simulink model "HIL_version22b"  (R2022b)
settings: Solver=ode3  StartTime=0.0  StopTime=inf  FixedStep=0.01  RelTol=1e-3  EnableMultiTasking=on
undefined symbols (not defined in the file): K
libraries: arduinolib x3, simulink_extras x2, arduinosensorlib x1
settings Model: SimulationMode=external  ExtModeTrigDuration=2  Creator=Shehab Abdo  LastModifiedBy=Shehab Abdo
settings SolverCC: AutoInsertRateTranBlk=on
settings OptimizationCC: ReuseModelBlockBuffer=on  EnhancedBackFolding=on  PassReuseOutputArgsAs=Individual arguments  ZeroExternalMemoryAtStartup=off  ZeroInternalMemoryAtStartup=off  MaxStackSize=64  OptimizeBlockOrder=speed  DifferentSizesBufferReuse=on  OptimizationCustomize=off  EfficientTunableParamExpr=on
settings DebuggingCC: MultiTaskRateTransMsg=warning  ParameterTunabilityLossMsg=error
settings HardwareCC: ProdBitPerInt=16  ProdBitPerPointer=16  ProdBitPerSizeT=16  ProdBitPerPtrDiffT=16  ProdLargestAtomicFloat=None  ProdWordSize=8  ProdHWDeviceType=Atmel->AVR
settings SFSimCC: MATLABDynamicMemAlloc=off
settings RTWCC: Description=Embedded Coder  SystemTargetFile=ert.tlc  HardwareBoard=Arduino Mega 2560  TLCOptions=-aInlineSetEventsForThisBaseRateFcn=TLC_FALSE -aSuppressMultiTaskScheduler=TLC_FALSE -aRateBasedStepFcn=1  TemplateMakefile=ert_default_tmf  Toolchain=Arduino AVR  BuildConfiguration=Faster Runs
settings CodeAppCC: ForceParamTrailComments=on  IgnoreCustomStorageClasses=off  OperatorAnnotations=on  SimulinkDataObjDesc=on  SFDataObjDesc=on  InsertBlockDesc=on
settings ERTTargetCC: SupportContinuousTime=on  SupportVariableSizeSignals=on  ExtModeTransport=3  ExtModeStaticAlloc=on  ExtModeAutomaticAllocSize=off  ExtModeStaticAllocSize=2048  ExtModeMexFile=ext_xcp  ExtModeIntrfLevel=Level2 - Open

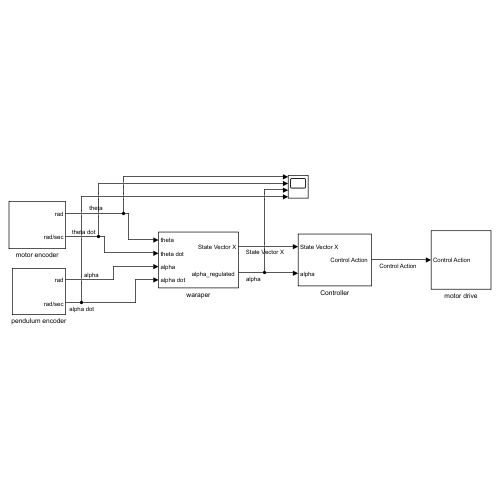
[thumbnail: Simulink's stored preview of the top-level diagram]
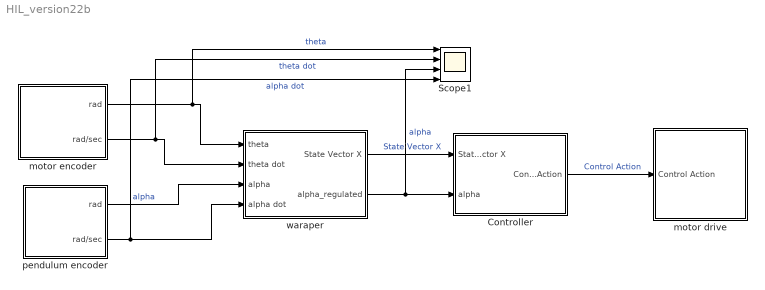
== system HIL_version22b ==
  Controller : Subsystem
  Scope1 : Scope  NumInputPorts=4
  motor drive : Subsystem
  motor encoder : Subsystem
  pendulum encoder : Subsystem
  waraper : Subsystem
  wires:
  Controller/1("Control Action ") -> motor drive/1(Control Action)  "Control Action"
  waraper/2("alpha_regulated ") -> Scope1/3, Controller/2(alpha)  "alpha"
  pendulum encoder/1(rad) -> waraper/3(alpha)  "alpha"
  motor encoder/2(rad/sec) -> Scope1/2, waraper/2(theta dot)  "theta dot"
  waraper/1(State Vector X) -> Controller/1(State Vector X)  "State Vector X"
  motor encoder/1(rad) -> Scope1/1, waraper/1(theta)  "theta"
  pendulum encoder/2(rad/sec) -> waraper/4(alpha dot), Scope1/4  "alpha dot"

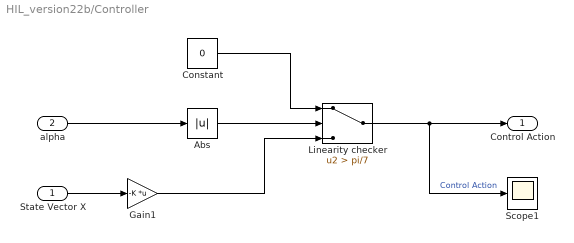
== system HIL_version22b/Controller ==
  State Vector X : Inport
  alpha : Inport  Port=2
  Abs : Abs  SaturateOnIntegerOverflow=off
  Constant : Constant  Value=0
  Gain1 : Gain  Gain=-K  Multiplication=Matrix(K*u)
  Linearity checker : Switch  Criteria=u2 > Threshold  Threshold=pi/7  SaturateOnIntegerOverflow=off  InputSameDT=off
  Scope1 : Scope
  "Control Action " : Outport
  wires:
  State Vector X/1 -> Gain1/1
  Constant/1 -> Linearity checker/1
  Linearity checker/1 -> "Control Action "/1, Scope1/1  "Control Action"
  Gain1/1 -> Linearity checker/3
  Abs/1 -> Linearity checker/2
  alpha/1 -> Abs/1

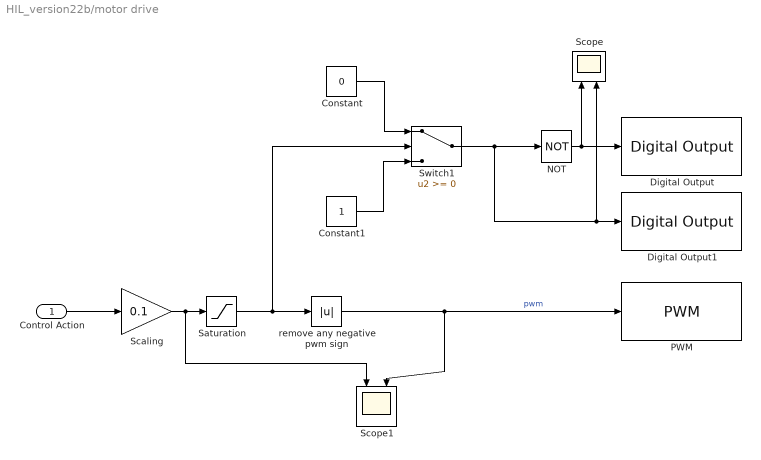
== system HIL_version22b/motor drive ==
  Control Action : Inport
  Constant : Constant  Value=0
  Constant1 : Constant
  Digital Output : arduinolib/Digital Output  pinNumber=7  Direction=output  blockPlatform=arduino
  Digital Output1 : arduinolib/Digital Output  pinNumber=8  Direction=output  blockPlatform=arduino
  NOT : Logic  Operator=NOT  IconShape=distinctive  AllPortsSameDT=off  OutDataTypeStr=boolean
  PWM : arduinolib/PWM  pinNumber=6  frequencyType=Default  desiredFrequency=490.2  achievableFrequency=490.2
  Saturation : Saturate  UpperLimit=255  LowerLimit=-255
  Scaling : Gain  Gain=0.1
  Scope : Scope  NumInputPorts=2
  Scope1 : Scope  NumInputPorts=2
  Switch1 : Switch  SaturateOnIntegerOverflow=off  InputSameDT=off
  remove any negative pwm sign : Abs  SaturateOnIntegerOverflow=off
  wires:
  remove any negative pwm sign/1 -> PWM/1, Scope1/2  "pwm"
  Saturation/1 -> Switch1/2, remove any negative pwm sign/1
  Constant/1 -> Switch1/1
  Control Action/1 -> Scaling/1
  Scaling/1 -> Scope1/1, Saturation/1
  Constant1/1 -> Switch1/3
  Switch1/1 -> Digital Output1/1, Scope/2, NOT/1
  NOT/1 -> Digital Output/1, Scope/1

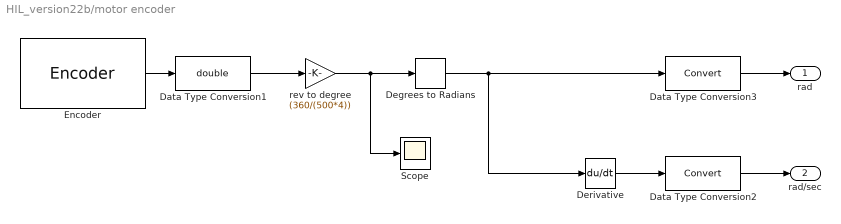
== system HIL_version22b/motor encoder ==
  Data Type Conversion1 : DataTypeConversion  OutDataTypeStr=double  SaturateOnIntegerOverflow=off  RndMeth=Floor
  Data Type Conversion2 : DataTypeConversion  SaturateOnIntegerOverflow=off  RndMeth=Floor
  Data Type Conversion3 : DataTypeConversion  SaturateOnIntegerOverflow=off  RndMeth=Floor
  Degrees to Radians : simulink_extras/Transformations/Degrees to Radians
  Derivative : Derivative
  Encoder : arduinosensorlib/Encoder  InputA=2  InputB=3  Mode=No reset  SampleTime=-1
  Scope : Scope
  rev to degree : Gain  Gain=(360/(500*4))
  rad : Outport
  rad/sec : Outport  Port=2
  wires:
  Derivative/1 -> Data Type Conversion2/1
  rev to degree/1 -> Scope/1, Degrees to Radians/1
  Degrees to Radians/1 -> Derivative/1, Data Type Conversion3/1
  Data Type Conversion3/1 -> rad/1
  Data Type Conversion2/1 -> rad/sec/1
  Data Type Conversion1/1 -> rev to degree/1
  Encoder/1 -> Data Type Conversion1/1

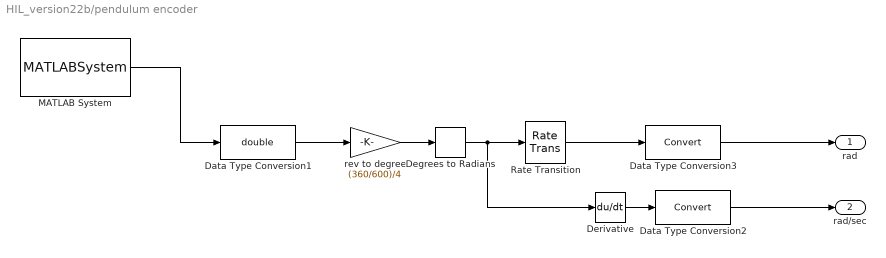
== system HIL_version22b/pendulum encoder ==
  Data Type Conversion1 : DataTypeConversion  OutDataTypeStr=double  SaturateOnIntegerOverflow=off  RndMeth=Floor
  Data Type Conversion2 : DataTypeConversion  SaturateOnIntegerOverflow=off  RndMeth=Floor
  Data Type Conversion3 : DataTypeConversion  SaturateOnIntegerOverflow=off  RndMeth=Floor
  Degrees to Radians : simulink_extras/Transformations/Degrees to Radians
  Derivative : Derivative
  MATLAB System : MATLABSystem  System=Encoder_arduino  Encoder=0  PinA=18  PinB=19  SampleTime=0.1
      mask Type: Encoder_arduino
      mask Display:
      | disp('Encoder');
      | port_label('output',1,'y');
  Rate Transition : RateTransition
  rev to degree : Gain  Gain=(360/600)/4
  rad : Outport
  rad/sec : Outport  Port=2
  wires:
  Data Type Conversion3/1 -> rad/1
  Data Type Conversion2/1 -> rad/sec/1
  Data Type Conversion1/1 -> rev to degree/1
  rev to degree/1 -> Degrees to Radians/1
  Derivative/1 -> Data Type Conversion2/1
  Degrees to Radians/1 -> Derivative/1, Rate Transition/1
  MATLAB System/1 -> Data Type Conversion1/1
  Rate Transition/1 -> Data Type Conversion3/1

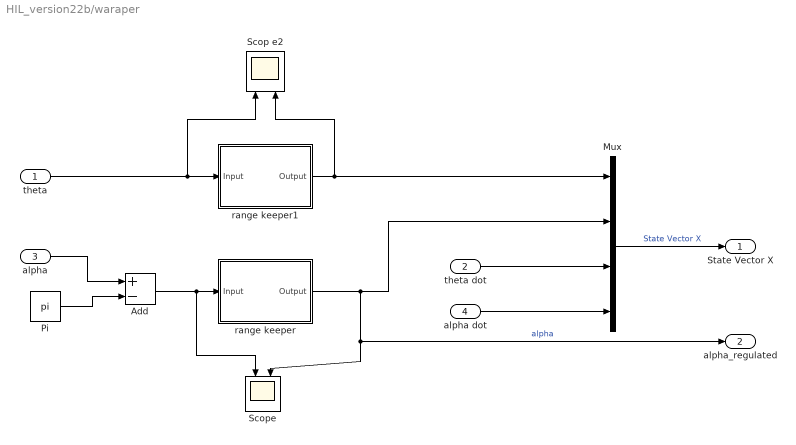
== system HIL_version22b/waraper ==
  theta : Inport
  theta dot : Inport  Port=2
  alpha : Inport  Port=3
  alpha dot : Inport  Port=4
  Add : Sum  Inputs=+-
  Mux : Mux
  Pi : Constant  Value=pi  OutDataTypeStr=Inherit: Inherit via back propagation
  Scop e2 : Scope  NumInputPorts=2
  Scope : Scope  NumInputPorts=2
  range keeper : Subsystem
  range keeper1 : Subsystem
  State Vector X : Outport
  "alpha_regulated " : Outport  Port=2
  wires:
  theta/1 -> range keeper1/1(Input), Scop e2/1
  Mux/1 -> State Vector X/1  "State Vector X"
  range keeper1/1(Output) -> Mux/1, Scop e2/2
  alpha dot/1 -> Mux/4
  Pi/1 -> Add/2
  Add/1 -> Scope/1, range keeper/1(Input)
  range keeper/1(Output) -> Mux/2, "alpha_regulated "/1, Scope/2  "alpha"
  alpha/1 -> Add/1
  theta dot/1 -> Mux/3

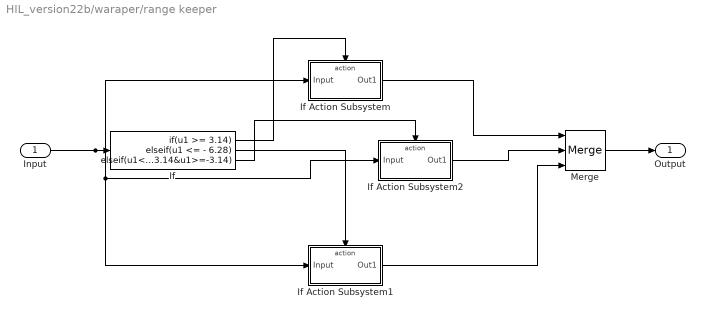
== system HIL_version22b/waraper/range keeper ==
  Input : Inport
  If : If  IfExpression=u1 >= 3.14  ElseIfExpressions=u1 <= - 6.28,u1<3.14&u1>=-3.14  ShowElse=off
  If Action Subsystem : Subsystem  TreatAsAtomicUnit=on
  If Action Subsystem1 : Subsystem  TreatAsAtomicUnit=on
  If Action Subsystem2 : Subsystem  TreatAsAtomicUnit=on
  Merge : Merge  Inputs=3
  Output : Outport
  wires:
  Merge/1 -> Output/1
  If Action Subsystem1/1(Out1) -> Merge/3
  If Action Subsystem/1(Out1) -> Merge/1
  If Action Subsystem2/1(Out1) -> Merge/2
  If/2 -> If Action Subsystem1/Action
  If/1 -> If Action Subsystem/Action
  Input/1 -> If Action Subsystem2/1(Input), If Action Subsystem1/1(Input), If Action Subsystem/1(Input), If/1
  If/3 -> If Action Subsystem2/Action

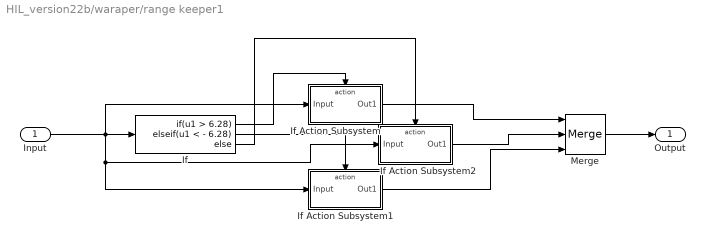
== system HIL_version22b/waraper/range keeper1 ==
  Input : Inport
  If : If  IfExpression=u1 > 6.28  ElseIfExpressions=u1 < - 6.28
  If Action Subsystem : Subsystem  TreatAsAtomicUnit=on
  If Action Subsystem1 : Subsystem  TreatAsAtomicUnit=on
  If Action Subsystem2 : Subsystem  TreatAsAtomicUnit=on
  Merge : Merge  Inputs=3
  Output : Outport
  wires:
  Input/1 -> If Action Subsystem2/1(Input), If Action Subsystem1/1(Input), If Action Subsystem/1(Input), If/1
  Merge/1 -> Output/1
  If Action Subsystem1/1(Out1) -> Merge/3
  If/1 -> If Action Subsystem/Action
  If Action Subsystem/1(Out1) -> Merge/1
  If/2 -> If Action Subsystem1/Action
  If/3 -> If Action Subsystem2/Action
  If Action Subsystem2/1(Out1) -> Merge/2

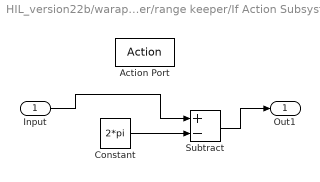
== system HIL_version22b/waraper/range keeper/If Action Subsystem ==
  Input : Inport
  Action Port : ActionPort  InitializeStates=reset  ActionPortLabel=if(u1 >= 3.14)
  Constant : Constant  Value=2*pi
  Subtract : Sum  Inputs=+-
  Out1 : Outport
  wires:
  Constant/1 -> Subtract/2
  Input/1 -> Subtract/1
  Subtract/1 -> Out1/1

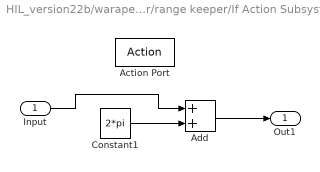
== system HIL_version22b/waraper/range keeper/If Action Subsystem1 ==
  Input : Inport
  Action Port : ActionPort  InitializeStates=reset  ActionPortLabel=elseif(u1 <= - 6.28)
  Add : Sum
  Constant1 : Constant  Value=2*pi
  Out1 : Outport
  wires:
  Constant1/1 -> Add/2
  Input/1 -> Add/1
  Add/1 -> Out1/1

== system HIL_version22b/waraper/range keeper/If Action Subsystem2 ==
  Input : Inport
  Action Port : ActionPort  ActionPortLabel=elseif(u1<3.14&u1>=-3.14)
  Out1 : Outport
  wires:
  Input/1 -> Out1/1

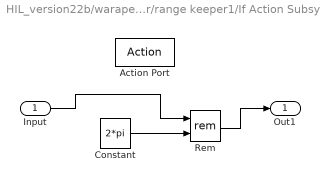
== system HIL_version22b/waraper/range keeper1/If Action Subsystem ==
  Input : Inport
  Action Port : ActionPort  ActionPortLabel=if(u1 > 6.28)
  Constant : Constant  Value=2*pi
  Rem : Math  Operator=rem  SignedPower=on
  Out1 : Outport
  wires:
  Constant/1 -> Rem/2
  Input/1 -> Rem/1
  Rem/1 -> Out1/1

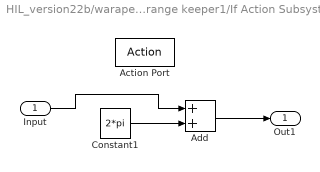
== system HIL_version22b/waraper/range keeper1/If Action Subsystem1 ==
  Input : Inport
  Action Port : ActionPort  ActionPortLabel=elseif(u1 < - 6.28)
  Add : Sum
  Constant1 : Constant  Value=2*pi
  Out1 : Outport
  wires:
  Constant1/1 -> Add/2
  Input/1 -> Add/1
  Add/1 -> Out1/1

== system HIL_version22b/waraper/range keeper1/If Action Subsystem2 ==
  Input : Inport
  Action Port : ActionPort  ActionPortLabel=else
  Out1 : Outport
  wires:
  Input/1 -> Out1/1
